simulink model "ECU_Durum_Makinesi"  (R2023a)
settings: Solver=ode3  StartTime=0.0  StopTime=100  FixedStep=0.01  RelTol=1e-3
undefined symbols (not defined in the file or in its folder): canChannel
libraries: canmsglib x6, canlib x1, slpidlib x1
settings Model: Creator=MEHMET  LastModifiedBy=MEHMET

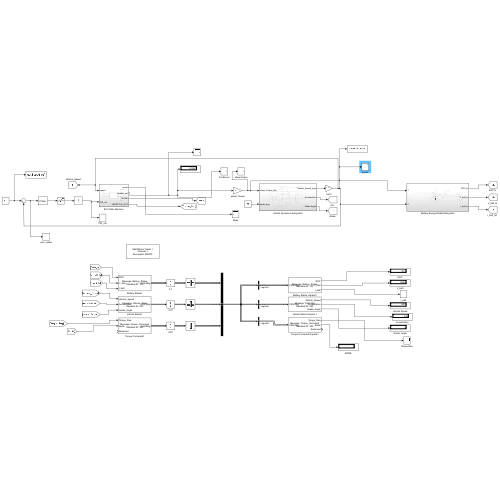
[thumbnail: Simulink's stored preview of the top-level diagram]
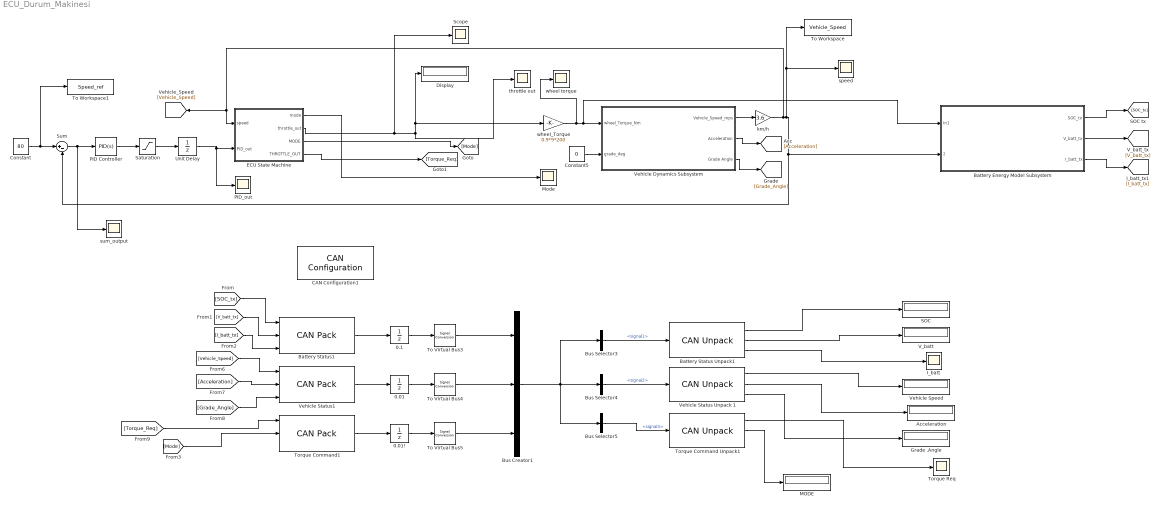
== system ECU_Durum_Makinesi ==
  0.01 : UnitDelay  InitialCondition=0.01  SampleTime=-1  HasFrameUpgradeWarning=on
  0.01! : UnitDelay  InitialCondition=0.1  SampleTime=-1  HasFrameUpgradeWarning=on
  0.1 : UnitDelay  InitialCondition=0.1  SampleTime=-1  HasFrameUpgradeWarning=on
  Acceleration : Display
  Battery Energy Model Subsystem : Subsystem
  Battery Status Unpack1 : canmsglib/CAN Unpack  MsgList=(none)  MsgName=Battery_Status  MsgIDType=Standard (11-bit identifier)  MsgIdentifier=100  MsgLength=8  SignalInfo={ 'SOC', '0', '16', 'LE', 'unsigned', 'Standard', '0', '0.1', '0', '-Inf', 'Inf'; 'V_batt', '16', '16', 'LE', 'unsigned', 'Standard', '0', '0.1', '0', '-Inf', 'Inf'; 'I_batt', '32', '16', 'LE', 'unsigned', 'Standard', '0', '0.01', '0', '-Inf', 'Inf' }  IDPort=off  TimestampPort=off  ErrorPort=off  RemotePort=off  LengthPort=off  StatusPort=off  ApplyMinMax=off
      settings: LibrarySourceBlock=canlib/CAN Unpack
  Battery Status1 : canmsglib/CAN Pack  MsgList=(none)  MsgName=Battery_Status  MsgIDType=Standard (11-bit identifier)  MsgIdentifier=100  MsgLength=8  Remote=off  ApplyMinMax=off  BusOutput=on  SignalInfo={ 'SOC', '0', '16', 'LE', 'unsigned', 'Standard', '0', '0.1', '0', '-Inf', 'Inf'; 'V_batt', '16', '16', 'LE', 'unsigned', 'Standard', '0', '0.1', '0', '-Inf', 'Inf'; 'I_batt', '32', '16', 'LE', 'unsigned', 'Standard', '0', '0.01', '0', '-Inf', 'Inf' }
      settings: LibrarySourceBlock=canlib/CAN Pack  DataFormat=manually specified signals
  Bus Creator1 : BusCreator  Inputs=3
  Bus Selector3 : BusSelector  OutputSignals=signal1
  Bus Selector4 : BusSelector  OutputSignals=signal2
  Bus Selector5 : BusSelector  OutputSignals=signal3
  CAN Configuration1 : canlib/CAN Configuration  BlockHandle=89.0004  Device=MathWorks Virtual 1 (Channel 1)  DeviceMenu=MathWorks Virtual 1 (Channel 1)  ObjConstructor=canChannel('MathWorks', 'Virtual 1', 1)  BusSpeed=500000  EnableBitParameters=off  AckMode=Normal
  Constant : Constant  Value=80
  Constant5 : Constant  Value=0
  Display : Display
  ECU State Machine : Subsystem
  Grade .Angle : Display
  I_batt : Scope
  MODE : Display
  Mode : Scope
  PID Controller : slpidlib/PID Controller  Controller=PID  Form=Parallel  TimeDomain=Continuous-time  UseExternalTs=off  SampleTime=-1  IntegratorMethod=Forward Euler  FilterMethod=Forward Euler  ControllerParametersSource=internal  P=5.6  I=0.1  UseKiTs=off  D=0.1  N=100  UseFilter=on  TunerSelectOption=Transfer Function Based (PID Tuner App)  InitialConditionSource=internal  InitialConditionForIntegrator=0  InitialConditionForFilter=0  DifferentiatorICPrevScaledInput=0  ExternalReset=none  TrackingMode=off  Kt=1  LimitOutput=off  SatLimitsSource=internal  UpperSaturationLimit=inf  LowerSaturationLimit=-inf  LinearizeAsGain=on  AntiWindupMode=none  Kb=1  LimitIntegrator=off  UpperIntegratorSaturationLimit=inf  LowerIntegratorSaturationLimit=-inf  POutMin=[]  POutMax=[]  IOutMin=[]  IOutMax=[]  DOutMin=[]  DOutMax=[]  NOutMin=[]  NOutMax=[]  SumOutMin=[]  SumOutMax=[]  SaturationOutMin=[]  SaturationOutMax=[]  PParamMin=[]  PParamMax=[]  IParamMin=[]  IParamMax=[]  DParamMin=[]  DParamMax=[]  NParamMin=[]  NParamMax=[]  KbParamMin=[]  KbParamMax=[]  KtParamMin=[]  KtParamMax=[]  KbOutMin=[]  KbOutMax=[]  KtOutMin=[]  KtOutMax=[]  IntegratorOutMin=[]  IntegratorOutMax=[]  FilterOutMin=[]  FilterOutMax=[]  SumI1OutMin=[]  SumI1OutMax=[]  SumI2OutMin=[]  SumI2OutMax=[]  SumI3OutMin=[]  SumI3OutMax=[]  SumI4OutMin=[]  SumI4OutMax=[]  SumDOutMin=[]  SumDOutMax=[]  DifferentiatorOutMin=[]  DifferentiatorOutMax=[]  FilterDiffOutCoefMin=[]  FilterDiffOutCoefMax=[]  ReciprocalOutMin=[]  ReciprocalOutMax=[]  SumDenOutMin=[]  SumDenOutMax=[]  SumNumOutMin=[]  SumNumOutMax=[]  DivideOutMin=[]  DivideOutMax=[]  UdiffTsProdOutMin=[]  UdiffTsProdOutMax=[]  NTsProdOutMin=[]  NTsProdOutMax=[]  UintegralTsProdOutMin=[]  UintegralTsProdOutMax=[]  UngainTsProdOutMin=[]  UngainTsProdOutMax=[]  ClampingZeroOutDataTypeStr=Inherit: Inherit via back propagation  ClampingZeroOutMin=[]  ClampingZeroOutMax=[]  FilterDenConstantOutDataTypeStr=Inherit: Inherit via back propagation  FilterDenConstantOutMin=[]  FilterDenConstantOutMax=[]  PCopyOutDataTypeStr=Inherit: Inherit via back propagation  PCopyOutMin=[]  PCopyOutMax=[]  NCopyOutDataTypeStr=Inherit: Inherit via back propagation  NCopyOutMin=[]  NCopyOutMax=[]  IntegratorContinuousStateAttributes=''  IntegratorStateMustResolveToSignalObject=off  IntegratorRTWStateStorageClass=Auto  FilterContinuousStateAttributes=''  FilterStateMustResolveToSignalObject=off  FilterRTWStateStorageClass=Auto  ParallelPVariant=InternalParameters  IdealPVariant=Disabled  IVariant=InternalParameters  DVariant=InternalParameters  IntegratorVariant=Continuous  SatVariant=Disabled  AWVariant=Passthrough  PCopyVariant=Disabled  TRVariant=Disabled  FdbkBlocksVariant=Forward  IdealPFdbkVariant=Disabled  SatFdbkVariant=Disabled  DerivativeFilterVariant=ContFilter  NVariant=InternalParameters  NCopyVariant=Disabled  FilterICVariant=InternalICsFilter  IntegratorICVariant=InternalICs  ExternalResetVariant=Disabled  TRSumVariant=Passthrough  SumFdbkVariant=Disabled  SumVariant=Sum_PID  TsampFilterVariant=InternalTs  TsampNgainVariant=Passthrough  TsampIntegralVariant=Disabled_SignalSpec  ExternalSaturationOutDataTypeStr=Inherit: Same as second input
  PID_out : Scope
  SOC : Display
  Saturation : Saturate  UpperLimit=1  LowerLimit=0
  Scope : Scope
  Sum : Sum  Inputs=|+-
  To Virtual Bus3 : SignalConversion  ConversionOutput=Nonvirtual bus  OverrideOpt=off
  To Virtual Bus4 : SignalConversion  ConversionOutput=Nonvirtual bus  OverrideOpt=off
  To Virtual Bus5 : SignalConversion  ConversionOutput=Nonvirtual bus  OverrideOpt=off
  To Workspace : ToWorkspace  VariableName=Vehicle_Speed  SaveFormat=Timeseries  SampleTime=-1
  To Workspace1 : ToWorkspace  VariableName=Speed_ref  SaveFormat=Timeseries  SampleTime=-1
  Torque Command Unpack1 : canmsglib/CAN Unpack  MsgList=(none)  MsgName=Torque_Command  MsgIDType=Standard (11-bit identifier)  MsgIdentifier=300  MsgLength=8  SignalInfo={ 'Torque_Req', '0', '32', 'LE', 'single', 'Standard', '0', '1', '0', '-Inf', 'Inf'; 'Mode', '32', '8', 'LE', 'unsigned', 'Standard', '0', '1', '0', '-Inf', 'Inf'; 'Reserved', '40', '8', 'LE', 'unsigned', 'Standard', '0', '1', '0', '-Inf', 'Inf' }  IDPort=off  TimestampPort=off  ErrorPort=off  RemotePort=off  LengthPort=off  StatusPort=off  ApplyMinMax=off
      settings: LibrarySourceBlock=canlib/CAN Unpack
  Torque Command1 : canmsglib/CAN Pack  MsgList=(none)  MsgName=Torque_Command  MsgIDType=Standard (11-bit identifier)  MsgIdentifier=300  MsgLength=8  Remote=off  ApplyMinMax=off  BusOutput=on  SignalInfo={ 'Torque_Req', '0', '32', 'LE', 'single', 'Standard', '0', '1', '0', '-Inf', 'Inf'; 'Mode', '32', '8', 'LE', 'unsigned', 'Standard', '0', '1', '0', '-Inf', 'Inf'; 'Reserved', '40', '8', 'LE', 'unsigned', 'Standard', '0', '1', '0', '-Inf', 'Inf' }
      settings: LibrarySourceBlock=canlib/CAN Pack  DataFormat=manually specified signals
  Torque Req : Scope
  Unit Delay : UnitDelay  SampleTime=0.01  HasFrameUpgradeWarning=on
  V_batt : Display
  Vehicle Dynamics Subsystem : Subsystem
  Vehicle Speed : Display
  Vehicle Status Unpack 1 : canmsglib/CAN Unpack  MsgList=(none)  MsgName=CAN Msg  MsgIDType=Standard (11-bit identifier)  MsgIdentifier=200  MsgLength=8  SignalInfo={ 'Vehicle_Speed', '0', '16', 'LE', 'unsigned', 'Standard', '0', '0.1', '0', '-Inf', 'Inf'; 'Acceleration', '16', '16', 'LE', 'unsigned', 'Standard', '0', '0.01', '0', '-Inf', 'Inf'; 'Grade_Angle', '32', '16', 'LE', 'unsigned', 'Standard', '0', '0.1', '0', '-Inf', 'Inf' }  IDPort=off  TimestampPort=off  ErrorPort=off  RemotePort=off  LengthPort=off  StatusPort=off  ApplyMinMax=off
      settings: LibrarySourceBlock=canlib/CAN Unpack
  Vehicle Status1 : canmsglib/CAN Pack  MsgList=(none)  MsgName=Vehicle_State  MsgIDType=Standard (11-bit identifier)  MsgIdentifier=200  MsgLength=8  Remote=off  ApplyMinMax=off  BusOutput=on  SignalInfo={ 'Vehicle_Speed', '0', '16', 'LE', 'unsigned', 'Standard', '0', '0.1', '0', '-Inf', 'Inf'; 'Acceleration', '16', '16', 'LE', 'unsigned', 'Standard', '0', '0.01', '0', '-Inf', 'Inf'; 'Grade_Angle', '32', '16', 'LE', 'unsigned', 'Standard', '0', '0.1', '0', '-Inf', 'Inf' }
      settings: LibrarySourceBlock=canlib/CAN Pack  DataFormat=manually specified signals
  km/h : Gain  Gain=3.6
  speed : Scope
  sum_output : Scope
  throttle out : Scope
  wheel torque : Scope
  wheel_Torque : Gain  Gain=0.9*9*200
  wires:
  Vehicle Status Unpack 1/1 -> Vehicle Speed/1
  Torque Command Unpack1/1 -> Torque Req/1
  Constant5/1 -> Vehicle Dynamics Subsystem/2(grade_deg)
  Bus Selector3/1 -> Battery Status Unpack1/1  "<signal1>"
  To Virtual Bus5/1 -> Bus Creator1/3
  [V_batt_tx] -> Battery Status1/2
  [I_batt_tx] -> Battery Status1/3
  Battery Energy Model Subsystem/3(I_batt_tx) -> [I_batt_tx]
  To Virtual Bus4/1 -> Bus Creator1/2
  Vehicle Status Unpack 1/2 -> Acceleration/1
  Battery Status Unpack1/2 -> V_batt/1
  [Vehicle_Speed] -> Vehicle Status1/1
  Battery Status Unpack1/3 -> I_batt/1
  Bus Selector4/1 -> Vehicle Status Unpack 1/1  "<signal2>"
  [SOC_tx] -> Battery Status1/1
  To Virtual Bus3/1 -> Bus Creator1/1
  Battery Energy Model Subsystem/1(SOC_tx) -> [SOC_tx]
  Torque Command1/1 -> 0.01!/1
  Battery Energy Model Subsystem/2(V_batt_tx) -> [V_batt_tx]
  [Torque_Req] -> Torque Command1/1
  Bus Creator1/1 -> Bus Selector5/1, Bus Selector3/1, Bus Selector4/1
  [Acceleration] -> Vehicle Status1/2
  Vehicle Status Unpack 1/3 -> Grade .Angle/1
  Vehicle Dynamics Subsystem/3(Grade Angle) -> [Grade_Angle]
  Bus Selector5/1 -> Torque Command Unpack1/1  "<signal3>"
  Vehicle Status1/1 -> 0.01/1
  [Grade_Angle] -> Vehicle Status1/3
  Battery Status Unpack1/1 -> SOC/1
  Vehicle Dynamics Subsystem/2(Acceleration) -> [Acceleration]
  Battery Status1/1 -> 0.1/1
  Vehicle Dynamics Subsystem/1(Vehicle_Speed_mps) -> km/h/1
  wheel_Torque/1 -> wheel torque/1, Vehicle Dynamics Subsystem/1(wheel_Torque_Nm), Battery Energy Model Subsystem/1(In1)
  Sum/1 -> sum_output/1, PID Controller/1
  km/h/1 -> [Vehicle_Speed], ECU State Machine/1(speed), Sum/2, Battery Energy Model Subsystem/2(2), To Workspace/1, speed/1
  PID Controller/1 -> Saturation/1
  ECU State Machine/1(mode) -> Mode/1
  Unit Delay/1 -> PID_out/1, ECU State Machine/2(PID_out)
  Constant/1 -> To Workspace1/1, Sum/1
  Saturation/1 -> Unit Delay/1
  0.1/1 -> To Virtual Bus3/1
  0.01/1 -> To Virtual Bus4/1
  0.01!/1 -> To Virtual Bus5/1
  ECU State Machine/3(MODE) -> [Mode]
  [Mode] -> Torque Command1/2
  Torque Command Unpack1/2 -> MODE/1
  ECU State Machine/2(throttle_out) -> Scope/1, throttle out/1, wheel_Torque/1, Display/1
  ECU State Machine/4(THROTTLE_OUT) -> [Torque_Req]

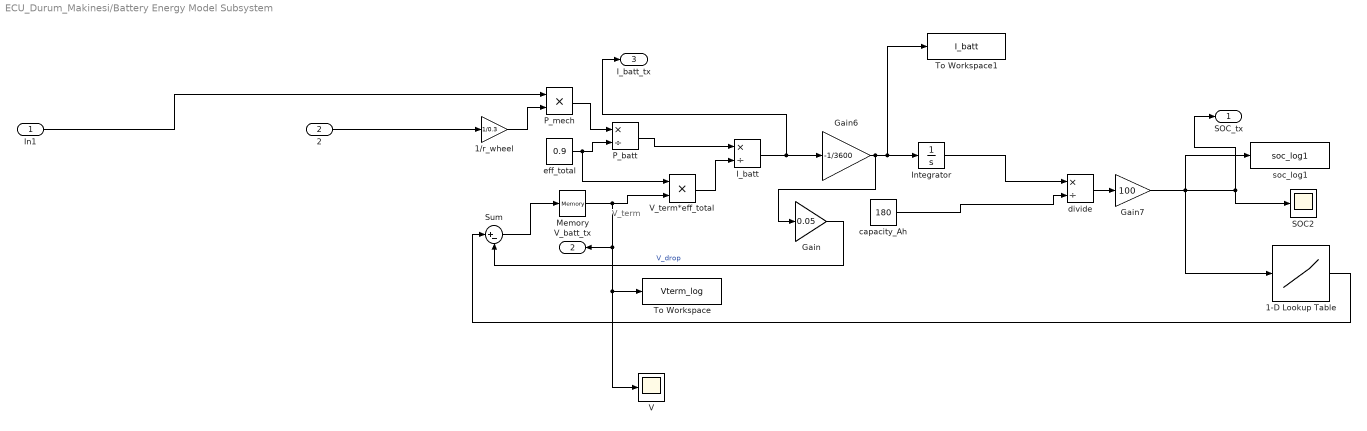
== system ECU_Durum_Makinesi/Battery Energy Model Subsystem ==
  note: V_term
  In1 : Inport
  2 : Inport  Port=2
  1-D Lookup Table : Lookup_n-D  NumberOfTableDimensions=1  BreakpointsForDimension1=[10 20 40 60 80 100]  Table=[325 332 342 350 356 360]  InternalRulePriority=Speed  RndMeth=Simplest
  1/r_wheel : Gain  Gain=1/0.3
  Gain : Gain  Gain=0.05
  Gain6 : Gain  Gain=-1/3600
  Gain7 : Gain  Gain=100
  I_batt : Product  Inputs=*/  RndMeth=Zero  SaturateOnIntegerOverflow=on
  Integrator : Integrator  InitialCondition=180
  Memory : Memory  InitialCondition=0.01
  P_batt : Product  Inputs=*/
  P_mech : Product
  SOC2 : Scope
  Sum : Sum  Inputs=|+-
  To Workspace : ToWorkspace  VariableName=Vterm_log  SampleTime=-1
  To Workspace1 : ToWorkspace  VariableName=I_batt  SampleTime=-1
  V : Scope
  V_term*eff_total : Product
  capacity_Ah : Constant  Value=180
  divide : Product  Inputs=*/  RndMeth=Zero  SaturateOnIntegerOverflow=on
  eff_total : Constant  Value=0.9
  soc_log1 : ToWorkspace  VariableName=soc_log1  SampleTime=-1
  SOC_tx : Outport
  V_batt_tx : Outport  Port=2
  I_batt_tx : Outport  Port=3
  wires:
  Integrator/1 -> divide/1
  P_batt/1 -> I_batt/1
  2/1 -> 1/r_wheel/1
  In1/1 -> P_mech/1
  capacity_Ah/1 -> divide/2
  divide/1 -> Gain7/1
  1/r_wheel/1 -> P_mech/2
  P_mech/1 -> P_batt/1
  eff_total/1 -> V_term*eff_total/1, P_batt/2
  Gain7/1 -> soc_log1/1, 1-D Lookup Table/1, SOC_tx/1, SOC2/1
  1-D Lookup Table/1 -> Sum/1
  Memory/1 -> V_batt_tx/1, V/1, To Workspace/1, V_term*eff_total/2
  Sum/1 -> Memory/1
  I_batt/1 -> I_batt_tx/1, Gain6/1
  Gain6/1 -> To Workspace1/1, Integrator/1, Gain/1
  Gain/1 -> Sum/2  "V_drop"
  V_term*eff_total/1 -> I_batt/2

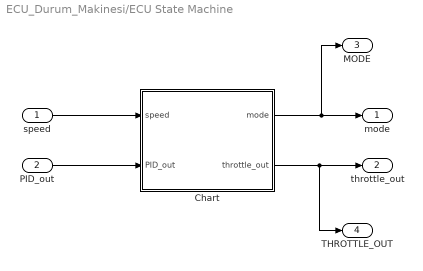
== system ECU_Durum_Makinesi/ECU State Machine ==
  speed : Inport
  PID_out : Inport  Port=2
  Chart : Stateflow chart  TreatAsAtomicUnit=on
  mode : Outport
  throttle_out : Outport  Port=2
  MODE : Outport  Port=3
  THROTTLE_OUT : Outport  Port=4
  wires:
  Chart/2(throttle_out) -> THROTTLE_OUT/1, throttle_out/1
  Chart/1(mode) -> MODE/1, mode/1
  PID_out/1 -> Chart/2(PID_out)
  speed/1 -> Chart/1(speed)

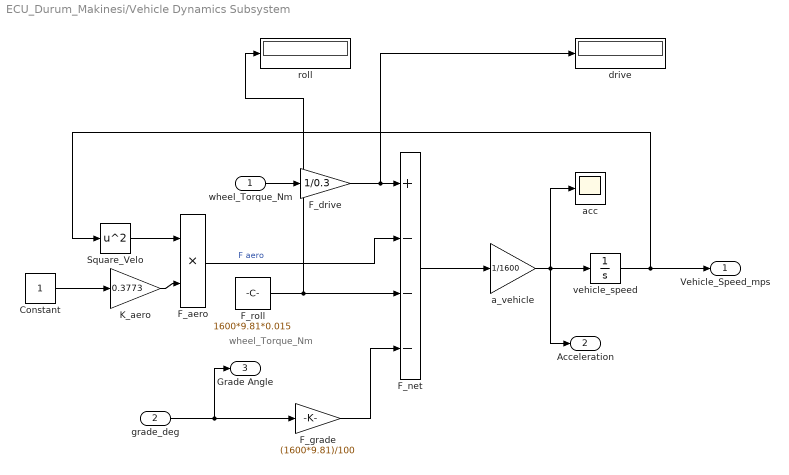
== system ECU_Durum_Makinesi/Vehicle Dynamics Subsystem ==
  note: wheel_Torque_Nm
  wheel_Torque_Nm : Inport
  grade_deg : Inport  Port=2
  Constant : Constant
  F_aero : Product
  F_drive : Gain  Gain=1/0.3
  F_grade : Gain  Gain=(1600*9.81)/100
  F_net : Sum  Inputs=+---
  F_roll : Constant  Value=1600*9.81*0.015
  K_aero : Gain  Gain=0.3773
  Square_Velo : Math  Operator=square
  a_vehicle : Gain  Gain=1/1600
  acc : Scope
  drive : Display
  roll : Display
  vehicle_speed : Integrator
  Vehicle_Speed_mps : Outport
  Acceleration : Outport  Port=2
  Grade Angle : Outport  Port=3
  wires:
  Square_Velo/1 -> F_aero/1
  grade_deg/1 -> Grade Angle/1, F_grade/1
  F_grade/1 -> F_net/4
  F_drive/1 -> drive/1, F_net/1
  F_aero/1 -> F_net/2  "F aero"
  a_vehicle/1 -> acc/1, Acceleration/1, vehicle_speed/1
  F_roll/1 -> F_net/3, roll/1
  Constant/1 -> K_aero/1
  K_aero/1 -> F_aero/2
  vehicle_speed/1 -> Square_Velo/1, Vehicle_Speed_mps/1
  wheel_Torque_Nm/1 -> F_drive/1
  F_net/1 -> a_vehicle/1

== stateflow chart ECU_Durum_Makinesi/ECU State Machine/Chart ==
  state Idle
    entry:
    mode=0;
    throttle_out=0;
  state Acceleration
    entry:
    mode=1;
    throttle_out=PID_out;
  state Cruise
    entry:
    mode=2
    throttle_out=PID_out;
  state Deceleration
    entry:
    mode=3;
    throttle_out=0;
  (default) -> Idle
  Idle -> Acceleration : [PID_out>0.05]
  Acceleration -> Cruise : [speed>= V_CRUISE - H]
  Cruise -> Deceleration : [speed>= V_CRUISE +H || PID_out<=0]
  Deceleration -> Idle [order 1] : [speed<=1]
  Deceleration -> Cruise [order 2] : [PID_out > 0.1 || speed < V_CRUISE - H]
  data: mode output size=1; throttle_out output size=1; speed input double size=1; PID_out input double size=1; H constant double size=1 =2; V_CRUISE constant double size=1 =80
  data mode settings: description=ECU operating mode (0=Idle, 1=Accel, 2=Cruise, 3=Decel
  data speed settings: description=Vehicle Speed Input fram Simulation
